simulink model "forwardConverter"  (R2021a)
settings: Solver=VariableStepAuto  StartTime=0.0  StopTime=10.0  RelTol=1e-3
model workspace (MAT data in the model file):
  Fs = Simulink.Parameter
  Fs.Value = 5000
  Fs.DataType = 'auto'
  Fs.Dimensions = [1 1]
  N1 = Simulink.Parameter
  N1.Value = 100
  N1.DataType = 'auto'
  N1.Dimensions = [1 1]
  N2 = Simulink.Parameter
  N2.Value = 200
  N2.DataType = 'auto'
  N2.Dimensions = [1 1]
  N3 = Simulink.Parameter
  N3.Value = 100
  N3.DataType = 'auto'
  N3.Dimensions = [1 1]
  Vin = Simulink.Parameter
  Vin.Value = 100
  Vin.DataType = 'auto'
  Vin.Dimensions = [1 1]
libraries: spsCurrentMeasurementLib x5, spsSeriesRLCBranchLib x4, spsDiodeLib x3, spsDCVoltageSourceLib x1, spsLinearTransformerLib x1, spsMeanLib x1, spsMosfetLib x1, spsVoltageMeasurementLib x1, spspowerguiLib x1
settings Model: Creator=User  LastModifiedBy=User

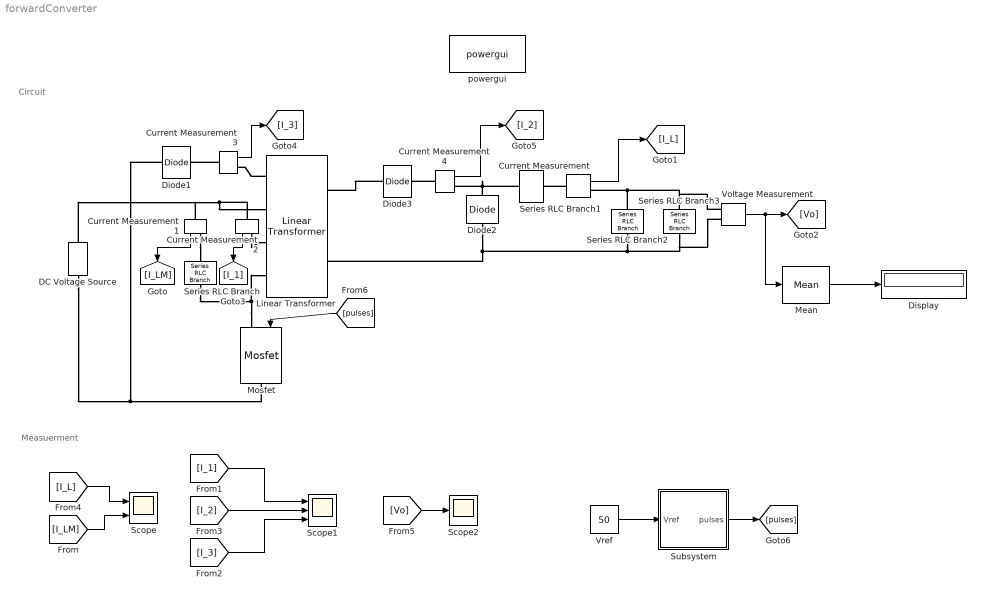
== system forwardConverter ==
  note: Circuit
  note: Measuerment
  Current Measurement{,1..4} (5 alike) : spsCurrentMeasurementLib/Current Measurement  PhasorSimulation=off  OutputType=Complex  PSBequivalent=0
  DC Voltage Source : spsDCVoltageSourceLib/DC Voltage Source  Amplitude=Vin  Measurements=None
  Diode1 : spsDiodeLib/Diode  Ron=0.001  Lon=0  Vf=0.8  IC=0  UseSnubber=0  Rs=500  Cs=250e-9  Measurements=off
  Diode2 : spsDiodeLib/Diode  Ron=0.001  Lon=0  Vf=0.8  IC=0  UseSnubber=0  Rs=500  Cs=250e-9  Measurements=off
  Diode3 : spsDiodeLib/Diode  Ron=0.001  Lon=0  Vf=0.8  IC=0  UseSnubber=0  Rs=500  Cs=250e-9  Measurements=off
  Display : Display
  Linear Transformer : spsLinearTransformerLib/Linear Transformer  UNITS=pu  NominalPower=[ 250e6 60 ]  winding1="[ N2 0  0 ]"  winding2="[ N3  0  0 ]"  ThreeWindings=on  winding3=[ N1 0 0 ]  RmLm=[ 500 500 ]  Measurements=None  DataType=off
  Mean : spsMeanLib/Mean  Freq=60  Vinit=0  Ts=0
  Mosfet : spsMosfetLib/Mosfet  Ron=0.1  Lon=0  Rd=0.01  Vfd=0  IC=0  Rs=1e5  Cs=inf  Measurements=off
  Scope : Scope  NumInputPorts=2
  Scope1 : Scope  NumInputPorts=3
  Scope2 : Scope
  Series RLC Branch : spsSeriesRLCBranchLib/Series RLC Branch  LConnTagsString=__new0  RConnTagsString=__new0  BranchType=L  Resistance=1  Inductance=1e-6  SetiL0=off  InitialCurrent=0  Capacitance=1e-6  Setx0=off  InitialVoltage=0  Measurements=None
  Series RLC Branch1 : spsSeriesRLCBranchLib/Series RLC Branch  LConnTagsString=__new0  RConnTagsString=__new0  BranchType=L  Resistance=1  Inductance=1e-2  SetiL0=off  InitialCurrent=0  Capacitance=1e-6  Setx0=off  InitialVoltage=0  Measurements=None
  Series RLC Branch2 : spsSeriesRLCBranchLib/Series RLC Branch  LConnTagsString=__new0  RConnTagsString=__new0  BranchType=C  Resistance=1  Inductance=1e-3  SetiL0=off  InitialCurrent=0  Capacitance=1e-3  Setx0=off  InitialVoltage=0  Measurements=None
  Series RLC Branch3 : spsSeriesRLCBranchLib/Series RLC Branch  LConnTagsString=__new0  RConnTagsString=__new0  BranchType=R  Resistance=10  Inductance=1e-3  SetiL0=off  InitialCurrent=0  Capacitance=1e-6  Setx0=off  InitialVoltage=0  Measurements=None
  Subsystem : Subsystem
  Voltage Measurement : spsVoltageMeasurementLib/Voltage Measurement  PhasorSimulation=off  OutputType=Complex  PSBequivalent=0
  Vref : Constant  Value=50
  powergui : spspowerguiLib/powergui  Priority=1  SimulationMode=Continuous  SampleTime=50e-6  frequency=60  Iterations=50  frequencyindice=0  Pbase=100e6  ErrMax=1e-4  UnitsV=kV  UnitsW=MW  buscounter=0  FunctionMessages=off  echomessages=off  EnableUseOfTLC=off  CurrentSourceSwitches=off  DisableSnubberDevices=off  DisableRonSwitches=off  DisableVfSwitches=off  DisplayEquations=off  AutomaticDiscreteSolvers=off  SolverType=Tustin/Backward Euler (TBE)  Interpol=off  ExternalGateDelay=off  methode=off  Ts=100  x0status=blocks  SPID=on  SwTol=0  HookPort=off  NonlinearTolerance=1e-4  nMaxIteration=100  ContinueOnMaxIteration=off  RestoreLinks=warning  ResistiveCurrentMeasurement=off  Frange=[0:2:500]  Ylog=off  Xlog=on  ShowGrid=off  save=off  variable=ZData  structure=0  ZoomFFT=off  StartTime=0.0  cycles=1  DisplayStyle=1  fundamental=60  FreqAxis=off  MaxFrequency=1000  frequencyindicesteady=1  RmsSteady=1  display=off
  wires:
  Current Measurement1/1 -> [I_LM]
  Current Measurement/1 -> [I_L]
  Voltage Measurement/1 -> Mean/1, [Vo]
  Current Measurement2/1 -> [I_1]
  Current Measurement3/1 -> [I_3]
  Current Measurement4/1 -> [I_2]
  [I_L] -> Scope/1
  [I_LM] -> Scope/2
  [I_1] -> Scope1/1
  [I_2] -> Scope1/2
  [I_3] -> Scope1/3
  [Vo] -> Scope2/1
  Subsystem/1(pulses) -> [pulses]
  [pulses] -> Mosfet/1
  Vref/1 -> Subsystem/1(Vref)
  Mean/1 -> Display/1
  connections:
  Current Measurement2/RConn1 -- Linear Transformer/RConn3
  Series RLC Branch/RConn1 -- Linear Transformer/RConn4 -- Mosfet/LConn1
  Current Measurement3/LConn1 -- Diode1/RConn1
  DC Voltage Source/LConn1 -- Diode1/LConn1 -- Mosfet/RConn1
  Diode3/LConn1 -- Linear Transformer/LConn1
  Diode2/RConn1 -- Series RLC Branch1/LConn1 -- Current Measurement4/RConn1
  Diode2/LConn1 -- Voltage Measurement/LConn2 -- Series RLC Branch3/RConn1 -- Series RLC Branch2/RConn1 -- Linear Transformer/LConn2
  Series RLC Branch2/LConn1 -- Voltage Measurement/LConn1 -- Series RLC Branch3/LConn1 -- Current Measurement/RConn1
  Current Measurement/LConn1 -- Series RLC Branch1/RConn1
  Current Measurement1/RConn1 -- Series RLC Branch/LConn1
  Current Measurement2/LConn1 -- DC Voltage Source/RConn1 -- Current Measurement1/LConn1 -- Linear Transformer/RConn2
  Linear Transformer/RConn1 -- Current Measurement3/RConn1
  Current Measurement4/LConn1 -- Diode3/RConn1

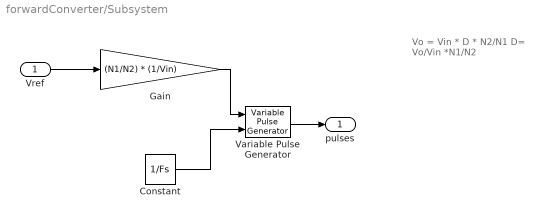
== system forwardConverter/Subsystem ==
  note: Vo = Vin * D * N2/N1
      | D= Vo/Vin *N1/N2
  Vref : Inport
  Constant : Constant  Value=1/Fs
  Gain : Gain  Gain=(N1/N2) * (1/Vin)
  Variable Pulse Generator : VariablePulseGenerator  SampleTime=0.1
  pulses : Outport
  wires:
  Variable Pulse Generator/1 -> pulses/1
  Vref/1 -> Gain/1
  Constant/1 -> Variable Pulse Generator/2
  Gain/1 -> Variable Pulse Generator/1
